simulink model "MOTORES"  (R2023b)
settings: Solver=VariableStepAuto  StartTime=0.0  StopTime=inf  RelTol=1e-3
libraries: arduinolib x2
settings Model: Creator=juanf  LastModifiedBy=juanf

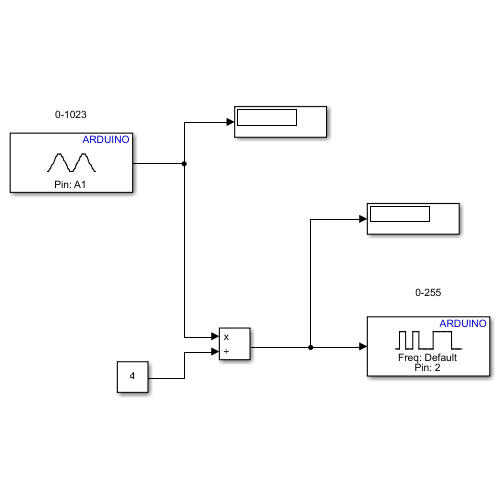
[thumbnail: Simulink's stored preview of the top-level diagram]
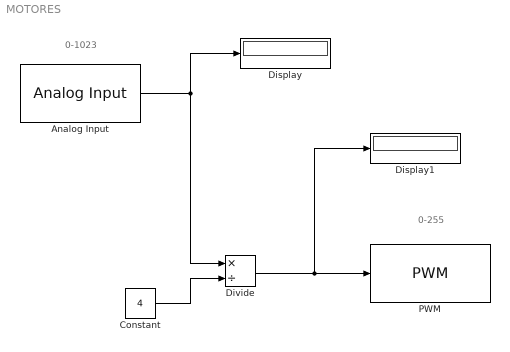
== system MOTORES ==
  note: 0-255
  note: 0-1023
  Analog Input : arduinolib/Analog Input  pinNumber=1  ReadResultsOnly=off  ConversionTriggerSource=Software  ExternalTriggerType=uint32( 0 )  OutputDataType=uint16  EnableConversionCompleteNotify=off  EnableOuputStatus=off  SampleTime=-1  blockPlatform=arduino
  Constant : Constant  Value=4
  Display : Display
  Display1 : Display
  Divide : Product  Inputs=*/
  PWM : arduinolib/PWM  pinNumber=2  frequencyType=Default  desiredFrequency=490.2  achievableFrequency=490.2
  wires:
  Analog Input/1 -> Display/1, Divide/1
  Divide/1 -> Display1/1, PWM/1
  Constant/1 -> Divide/2
